simulink model "Problem1"  (R2020a)
settings: Solver=VariableStepAuto  StartTime=0.0  StopTime=10.0  RelTol=1e-3
settings Model: Creator=sreeram  LastModifiedBy=sreeram

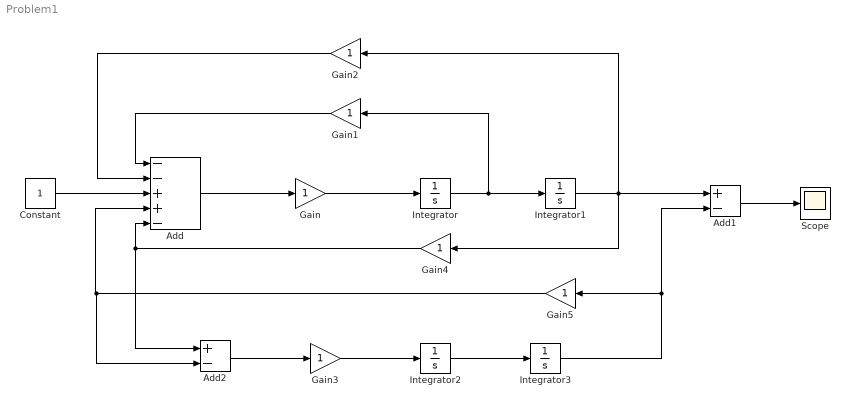
== system Problem1 ==
  Add : Sum  Inputs=--++-
  Add1 : Sum  Inputs=+-
  Add2 : Sum  Inputs=+-
  Constant : Constant
  Gain{,1..5} (6 alike) : Gain
  Integrator{,1..3} (4 alike) : Integrator
  Scope : Scope
  wires:
  Add/1 -> Gain/1
  Gain/1 -> Integrator/1
  Integrator/1 -> Gain1/1, Integrator1/1
  Integrator1/1 -> Gain2/1, Add1/1, Gain4/1
  Add1/1 -> Scope/1
  Constant/1 -> Add/3
  Gain1/1 -> Add/1
  Gain2/1 -> Add/2
  Add2/1 -> Gain3/1
  Gain3/1 -> Integrator2/1
  Integrator2/1 -> Integrator3/1
  Gain5/1 -> Add2/2, Add/4
  Integrator3/1 -> Gain5/1, Add1/2
  Gain4/1 -> Add2/1, Add/5
